simulink model "Pendulum02"  (R2018a)
settings: Solver=ode15s  StartTime=0.0  StopTime=5  MaxStep=0.001  RelTol=1e-3  EnableMultiTasking=on
values from neighbouring files (symbols this model uses):
  a = 1 / muscle_width^2    (= 3.1887755102)    [OldCodeForComparison.m]    (also in Parameters02.m)
  A0 = 0.2741    [OldCodeForComparison.m]    (also in Parameters02.m)
  A1 = -0.0627    [OldCodeForComparison.m]    (also in Parameters02.m)
  a_rel = 0.41    [OldCodeForComparison.m]    (also in Parameters02.m)
  alpha_a = 0.3 * 5/9    (= 0.166666666667)    [OldCodeForComparison.m]    (also in Parameters02.m)
  alpha_theta = 0.0    (= 0)    [OldCodeForComparison.m]    (also in Parameters02.m)
  alpha_v = 3.0 * 5/9    (= 1.66666666667)    [OldCodeForComparison.m]    (also in Parameters02.m)
  b_rel = 5.2    [OldCodeForComparison.m]    (also in Parameters02.m)
  d_l_CE = 0.06    [OldCodeForComparison.m]    (also in Parameters02.m)
  d_theta = 0.06    [OldCodeForComparison.m]    (also in Parameters02.m)
  d_thetaDot = 0.12    [OldCodeForComparison.m]    (also in Parameters02.m)
  d_thetaTwoDot = 0.12    [OldCodeForComparison.m]    (also in Parameters02.m)
  d_v_CE = 0.03    [OldCodeForComparison.m]    (also in Parameters02.m)
  F_max = 1.0e+04 * (0.5991 + 0.2996)    (= 8987)    [OldCodeForComparison.m]    (also in Parameters02.m)
  h_com = 1    [Parameters02.m]
  K_l = 1.0    (= 1)    [OldCodeForComparison.m]    (also in Parameters02.m)
  K_SE = 1.8e+05    (= 180000)    [OldCodeForComparison.m]    (also in Parameters02.m)
  K_v = 0.3    [OldCodeForComparison.m]    (also in Parameters02.m)
  l_CE_init = l_MTC - l_SE    [calculateMuscleEquilibriumState.m]
  l_CE_opt = 0.055    [OldCodeForComparison.m]    (also in Parameters02.m)
  l_SE_0 = 0.2356    [OldCodeForComparison.m]    (also in Parameters02.m)
  lambda_init = l_CE_init - 1 / K_l * STIM_init    [calculateMuscleEquilibriumState.m]
  m_body = 80    [Parameters02.m]
  muscle_c = 1.3700e-04    (= 0.000137)    [OldCodeForComparison.m]    (also in Parameters02.m)
  muscle_eta = 52700    [OldCodeForComparison.m]    (also in Parameters02.m)
  muscle_k = 2.9    [OldCodeForComparison.m]    (also in Parameters02.m)
  muscle_m = 11.3    [OldCodeForComparison.m]    (also in Parameters02.m)
  muscle_q0 = 0.005    [OldCodeForComparison.m]    (also in Parameters02.m)
  q_0 = 5e-03    (= 0.005)    [OldCodeForComparison.m]    (also in Parameters02.m)
  q_crit = 0.03    [OldCodeForComparison.m]    (also in Parameters02.m)
  theta_init = -0.05    [OldCodeForComparison.m]    (also in Parameters02.m)
undefined symbols (not defined in the file or in its folder): X, Y, Z
libraries: sm_lib x10, nesl_utility x9
settings Model: Creator=reimajbi  LastModifiedBy=reimajbi
settings DataIOCC: LimitDataPoints=on
settings OptimizationCC: LifeSpan=inf
settings DebuggingCC: AllowSymbolicDim=off  SFUnexpectedBacktrackingDiag=warning  SFNoUnconditionalDefaultTransitionDiag=warning  SFExecutionAtInitializationDiag=none
settings CodeAppCC: StateflowObjectComments=on
settings GRTTargetCC: TargetLangStandard=C89/C90 (ANSI)  GeneratePreprocessorConditionals=Disable all
settings ConfigComp: CovMetricSettings=dw  CovHtmlReporting=on  CovSaveCumulativeToWorkspaceVar=on  CovSaveSingleToWorkspaceVar=on  CovExternalEMLEnable=off  CovSFcnEnable=off
settings SimscapeCC: SimscapeNominalValues="[{\"value\":\"10\",\"unit\":\"V\"},{\"value\":\"1\",\"unit\":\"A\"},{\"value\":\"10\",\"unit\":\"N*m\"},{\"value\":\"10\",\"unit\":\"bar\"},{\"value\":\"100\",\"unit\":\"kJ/kg\"},{\"value\":\"1\",\"unit\":\"kW\"},{\"value\":\"300\",\"unit\":\"K\"},{\"value\":\"100\",\"unit\":\"cm^3/s\"},{\"value\":\"1\",\"unit\":\"kN\"},{\"value\":\"1\",\"unit\":\"g/cm^3\"},{\"value\":\"1\",\"unit\":\"l\"},{\"value\":\"1\",\"unit\":\"cm^2\"},{\"value\":\"60\",\"unit\":\"Hz\"}]"  SimscapeLogType=all  SimscapeLogDataHistory=10000
settings ConfigurationSet: Description=SimMechanics 2G

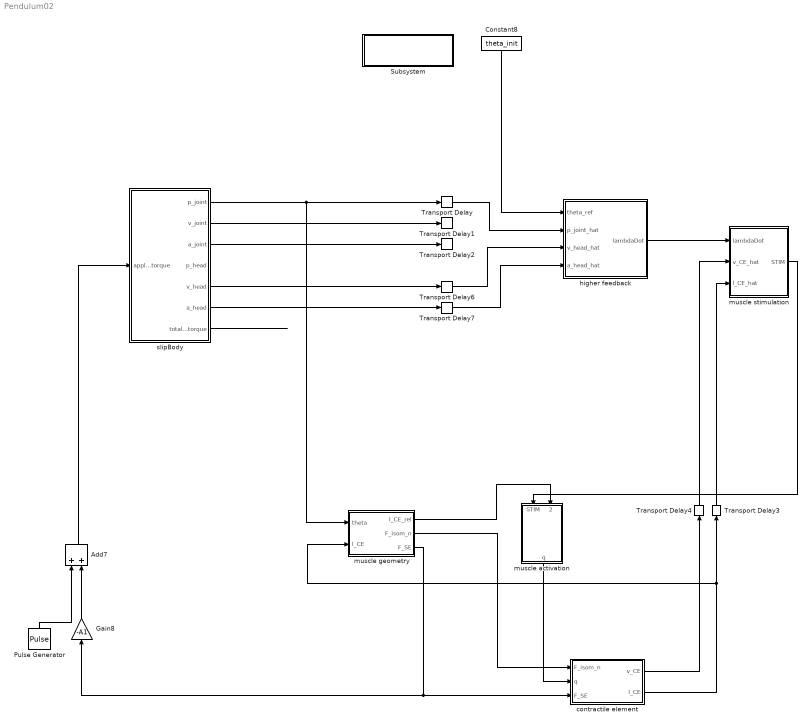
== system Pendulum02 ==
  Add7 : Sum
  Constant8 : Constant  Value=theta_init
  Gain8 : Gain  Gain=-A1
  Pulse Generator : DiscretePulseGenerator  PulseType=Time based  Amplitude=-50  Period=100  PulseWidth=0.2  PhaseDelay=0.1
  Subsystem : Subsystem
      settings: OpenFcn=open_system('sm_lib')
      mask Display: disp(sprintf('Open Simscape Multibody\nLibrary'));
  Transport Delay : TransportDelay  DelayTime=d_theta  InitialOutput=theta_init
  Transport Delay1 : TransportDelay  DelayTime=d_thetaDot
  Transport Delay2 : TransportDelay  DelayTime=d_thetaTwoDot
  Transport Delay3 : TransportDelay  DelayTime=d_l_CE  InitialOutput=l_CE_init
  Transport Delay4 : TransportDelay  DelayTime=d_v_CE
  Transport Delay6 : TransportDelay  DelayTime=d_thetaDot
  Transport Delay7 : TransportDelay  DelayTime=d_thetaTwoDot
  contractile element : Subsystem
  higher feedback : Subsystem
  muscle activation : Subsystem
  muscle geometry : Subsystem
  muscle stimulation : Subsystem
  slipBody : Subsystem  TreatAsAtomicUnit=on
  wires:
  Pulse Generator/1 -> Add7/1
  Gain8/1 -> Add7/2
  contractile element/1(v_CE) -> Transport Delay4/1
  contractile element/2(l_CE) -> muscle geometry/2(l_CE), Transport Delay3/1
  muscle activation/1(q) -> contractile element/2(q)
  Constant8/1 -> higher feedback/1(theta_ref)
  Transport Delay/1 -> higher feedback/2(p_joint_hat)
  Transport Delay6/1 -> higher feedback/3(v_head_hat)
  Transport Delay7/1 -> higher feedback/4(a_head_hat)
  higher feedback/1(lambdaDot) -> muscle stimulation/1(lambdaDot)
  Transport Delay4/1 -> muscle stimulation/2(v_CE_hat)
  Transport Delay3/1 -> muscle stimulation/3(l_CE_hat)
  muscle stimulation/1(STIM) -> muscle activation/1(STIM)
  muscle geometry/3(F_SE) -> Gain8/1, contractile element/3(F_SE)
  muscle geometry/1(l_CE_rel) -> muscle activation/2(l_CE_rel)
  muscle geometry/2(F_isom_n) -> contractile element/1(F_isom_n)
  slipBody/1(p_joint) -> muscle geometry/1(theta), Transport Delay/1
  Add7/1 -> slipBody/1(applied_torque)
  slipBody/2(v_joint) -> Transport Delay1/1
  slipBody/3(a_joint) -> Transport Delay2/1
  slipBody/5(v_head) -> Transport Delay6/1
  slipBody/6(a_head) -> Transport Delay7/1
  slipBody/7(total_torque) -> ?

== system Pendulum02/Subsystem ==

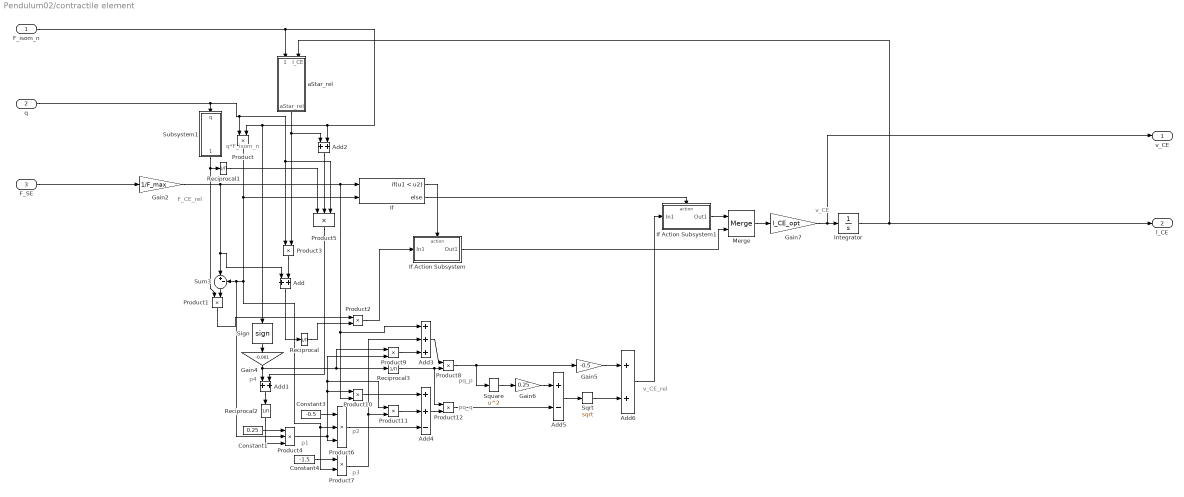
== system Pendulum02/contractile element ==
  note: v_CE_rel
  note: pq_q
  note: F_CE_rel
  note: p3
  note: p2
  note: q*F_isom_n
  note: p1
  note: p4
  note: pq_p
  note: v_CE
  F_isom_n : Inport
  q : Inport  Port=2
  F_SE : Inport  Port=3
  Add{,1..2,6} (4 alike) : Sum
  Add3 : Sum  Inputs=+++
  Add4 : Sum  Inputs=++-
  Add5 : Sum  Inputs=+-
  Constant1 : Constant  Value=0.25
  Constant3 : Constant  Value=-0.5
  Constant4 : Constant  Value=-1.5
  Gain2 : Gain  Gain=1/F_max
  Gain4 : Gain  Gain=-0.001
  Gain5 : Gain  Gain=-0.5
  Gain6 : Gain  Gain=0.25
  Gain7 : Gain  Gain=l_CE_opt
  If : If  NumInputs=2  IfExpression=u1 < u2
  If Action Subsystem : Subsystem  TreatAsAtomicUnit=on
  If Action Subsystem1 : Subsystem  TreatAsAtomicUnit=on
  Integrator : Integrator  InitialCondition=l_CE_init
  Merge : Merge
  Product{,1..3,7..12} (10 alike) : Product
  Product4 : Product  Inputs=3
  Product5 : Product  Inputs=3
  Product6 : Product  Inputs=3
  Reciprocal{,1..3} (4 alike) : Product  Inputs=/
  Sign : Signum
  Sqrt : Sqrt  SaturateOnIntegerOverflow=on
  Square : Math  Operator=square  SaturateOnIntegerOverflow=on
  Subsystem1 : Subsystem
  Sum3 : Sum  Inputs=|+-
  aStar_rel : Subsystem
  v_CE : Outport
  l_CE : Outport  Port=2
  wires:
  Sqrt/1 -> Add6/2
  Product1/1 -> Product2/1
  Add5/1 -> Sqrt/1
  Product10/1 -> Add4/1
  Constant1/1 -> Product4/1
  Gain6/1 -> Add5/1
  Add3/1 -> Product8/1
  Product5/1 -> Add1/2
  Product9/1 -> Add3/3
  Square/1 -> Gain6/1
  Add4/1 -> Product12/2
  F_SE/1 -> Gain2/1
  Reciprocal1/1 -> Product5/1
  Add2/1 -> Product5/2
  Reciprocal/1 -> Product2/2
  Product3/1 -> Add/2
  If Action Subsystem1/1(Out1) -> Merge/1
  Add1/1 -> Reciprocal2/1
  Sign/1 -> Gain4/1
  Product7/1 -> Add3/2, Product11/2
  Reciprocal3/1 -> Product12/1, Product8/2
  If/1 -> If Action Subsystem/Action
  Product2/1 -> If Action Subsystem/1(In1)
  Product11/1 -> Add4/2
  Gain4/1 -> Product9/1, Reciprocal3/1, Add1/1
  Add6/1 -> If Action Subsystem1/1(In1)
  Add/1 -> Reciprocal/1
  Product12/1 -> Add5/2
  Subsystem1/1(bStar_rel) -> Reciprocal1/1, Product1/1
  q/1 -> Product5/3, Product3/1, Product/1, Subsystem1/1(q)
  Gain7/1 -> v_CE/1, Integrator/1
  Constant4/1 -> Product7/1
  Gain5/1 -> Add6/1
  Product8/1 -> Square/1, Gain5/1
  Gain2/1 -> Sum3/1, Add/1, If/1, Add3/1, Product10/2
  Product4/1 -> Product10/1, Product11/1, Product9/2, Product6/3
  If/2 -> If Action Subsystem1/Action
  Integrator/1 -> l_CE/1, aStar_rel/2(l_CE)
  Sum3/1 -> Product1/2
  aStar_rel/1(aStar_rel) -> Add2/1, Product3/2
  If Action Subsystem/1(Out1) -> Merge/2
  Product6/1 -> Add4/3
  Reciprocal2/1 -> Product4/3
  F_isom_n/1 -> aStar_rel/1(F_isom_n), Sign/1, Product/2, Add2/2
  Constant3/1 -> Product6/1
  Merge/1 -> Gain7/1
  Product/1 -> Product7/2, Product6/2, Product4/2, Sum3/2, If/2

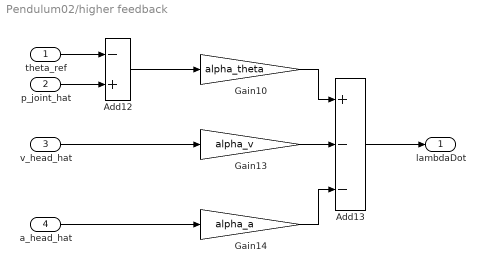
== system Pendulum02/higher feedback ==
  theta_ref : Inport
  p_joint_hat : Inport  Port=2
  v_head_hat : Inport  Port=3
  a_head_hat : Inport  Port=4
  Add12 : Sum  Inputs=-+
  Add13 : Sum  Inputs=+--
  Gain10 : Gain  Gain=alpha_theta
  Gain13 : Gain  Gain=alpha_v
  Gain14 : Gain  Gain=alpha_a
  lambdaDot : Outport
  wires:
  Add13/1 -> lambdaDot/1
  a_head_hat/1 -> Gain14/1
  v_head_hat/1 -> Gain13/1
  Gain10/1 -> Add13/1
  Gain14/1 -> Add13/3
  Gain13/1 -> Add13/2
  p_joint_hat/1 -> Add12/2
  theta_ref/1 -> Add12/1
  Add12/1 -> Gain10/1

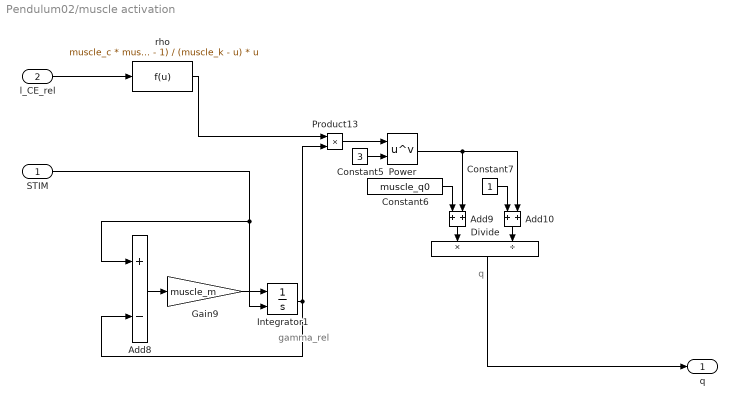
== system Pendulum02/muscle activation ==
  note: gamma_rel
  note: q
  STIM : Inport
  l_CE_rel : Inport  Port=2
  Add10 : Sum
  Add8 : Sum  Inputs=+-
  Add9 : Sum
  Constant5 : Constant  Value=3
  Constant6 : Constant  Value=muscle_q0
  Constant7 : Constant
  Divide : Product  Inputs=*/
  Gain9 : Gain  Gain=muscle_m
  Integrator1 : Integrator  InitialConditionSource=external  InitialCondition=0.038159574513235
  Power : Math  Operator=pow  SaturateOnIntegerOverflow=on
  Product13 : Product
  rho : Fcn  Expr=muscle_c * muscle_eta * (muscle_k - 1) / (muscle_k - u) * u
  q : Outport
  wires:
  l_CE_rel/1 -> rho/1
  Divide/1 -> q/1
  Constant7/1 -> Add10/1
  Product13/1 -> Power/1
  Constant5/1 -> Power/2
  Gain9/1 -> Integrator1/1
  Constant6/1 -> Add9/1
  Integrator1/1 -> Product13/2, Add8/2
  rho/1 -> Product13/1
  Add9/1 -> Divide/1
  Add10/1 -> Divide/2
  STIM/1 -> Integrator1/2, Add8/1
  Power/1 -> Add9/2, Add10/2
  Add8/1 -> Gain9/1

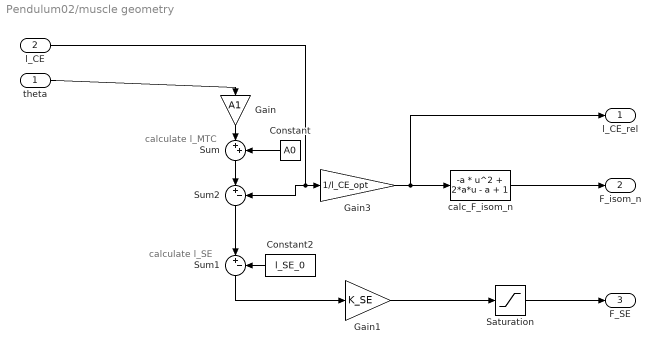
== system Pendulum02/muscle geometry ==
  note: calculate l_MTC
  note: calculate l_SE
  theta : Inport
  l_CE : Inport  Port=2
  Constant : Constant  Value=A0
  Constant2 : Constant  Value=l_SE_0
  Gain : Gain  Gain=A1
  Gain1 : Gain  Gain=K_SE
  Gain3 : Gain  Gain=1/l_CE_opt
  Saturation : Saturate  UpperLimit=inf  LowerLimit=0
  Sum : Sum  Inputs=|++
  Sum1 : Sum  Inputs=|+-
  Sum2 : Sum  Inputs=|+-
  calc_F_isom_n : Fcn  Expr=-a * u^2 + 2*a*u - a + 1
  l_CE_rel : Outport
  F_isom_n : Outport  Port=2
  F_SE : Outport  Port=3
  wires:
  calc_F_isom_n/1 -> F_isom_n/1
  Gain1/1 -> Saturation/1
  Constant/1 -> Sum/2
  Sum/1 -> Sum2/1
  Constant2/1 -> Sum1/2
  l_CE/1 -> Sum2/2, Gain3/1
  Gain3/1 -> l_CE_rel/1, calc_F_isom_n/1
  Sum1/1 -> Gain1/1
  Gain/1 -> Sum/1
  theta/1 -> Gain/1
  Saturation/1 -> F_SE/1
  Sum2/1 -> Sum1/1

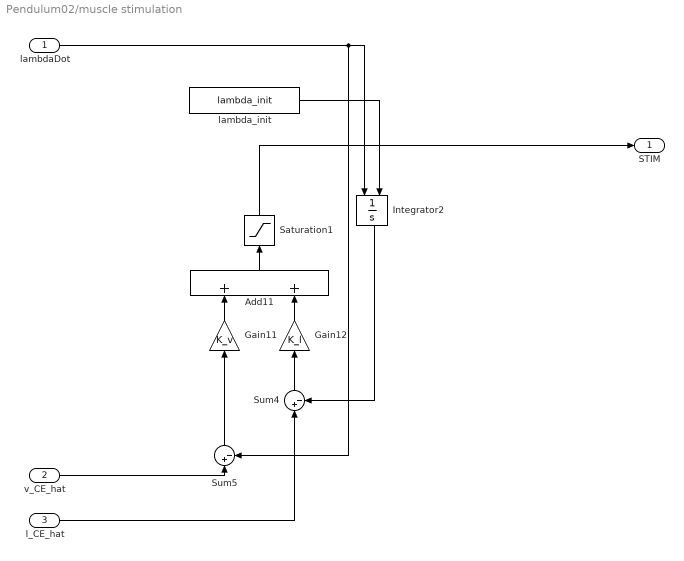
== system Pendulum02/muscle stimulation ==
  lambdaDot : Inport
  v_CE_hat : Inport  Port=2
  l_CE_hat : Inport  Port=3
  Add11 : Sum
  Gain11 : Gain  Gain=K_v
  Gain12 : Gain  Gain=K_l
  Integrator2 : Integrator  InitialConditionSource=external  InitialCondition=0.038159574513235
  Saturation1 : Saturate  UpperLimit=1  LowerLimit=0
  Sum4 : Sum  Inputs=|+-
  Sum5 : Sum  Inputs=|+-
  lambda_init : Constant  Value=lambda_init
  STIM : Outport
  wires:
  Saturation1/1 -> STIM/1
  l_CE_hat/1 -> Sum4/1
  lambda_init/1 -> Integrator2/2
  Sum4/1 -> Gain12/1
  Gain12/1 -> Add11/2
  Sum5/1 -> Gain11/1
  lambdaDot/1 -> Integrator2/1, Sum5/2
  Gain11/1 -> Add11/1
  v_CE_hat/1 -> Sum5/1
  Add11/1 -> Saturation1/1
  Integrator2/1 -> Sum4/2

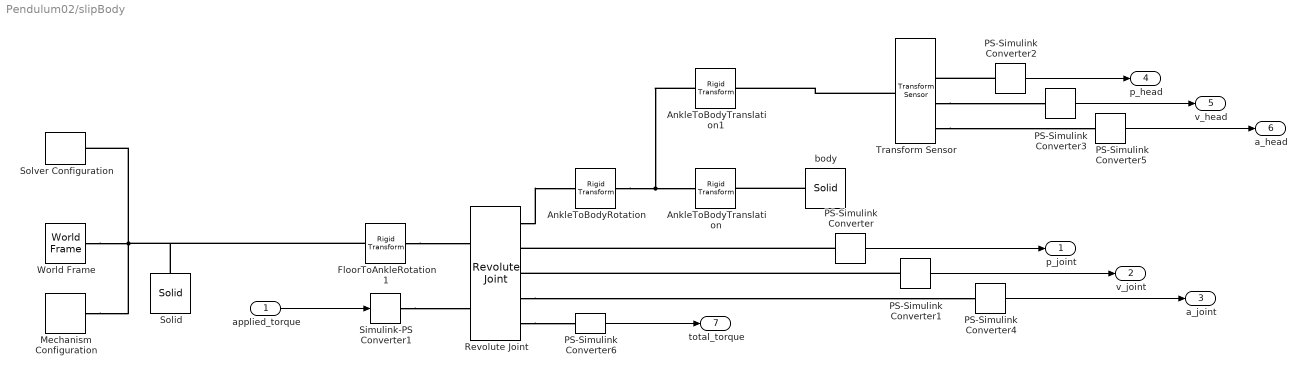
== system Pendulum02/slipBody ==
  applied_torque : Inport
  AnkleToBodyRotation : sm_lib/Frames and Transforms/Rigid Transform  TranslationMethod=None  TranslationStandardOffset=0  TranslationLengthUnit=m  TranslationStandardAxis=+Z  TranslationCartesianOffset=[0 0 0]  TranslationROffset=0  TranslationROffsetUnits=m  TranslationZOffset=0  TranslationZOffsetUnits=m  TranslationThetaOffset=0  TranslationThetaOffsetUnits=deg  RotationMethod=AlignedAxes  RotationAngleUnits=deg  RotationStandardAxis=+Z  RotationAngle=0.0  RotationArbitraryAxis=[0 0 1]  FollAlignAxisA=+Z  BaseAlignAxisA=+X  FollAlignAxisB=+Y  BaseAlignAxisB=+Z  RotationSequenceAxes=FollowerAxes  RotationSequence=XYX  RotationSequenceAngles=[0 0 0]  RotationSequenceAnglesUnits=deg  RotationMatrix=[1 0 0; 0 1 0; 0 0 1]
  AnkleToBodyTranslation : sm_lib/Frames and Transforms/Rigid Transform  TranslationMethod=StandardAxis  TranslationStandardOffset=h_com  TranslationLengthUnit=m  TranslationStandardAxis=+Z  TranslationCartesianOffset=[0 0 0]  TranslationROffset=0  TranslationROffsetUnits=m  TranslationZOffset=0  TranslationZOffsetUnits=m  TranslationThetaOffset=0  TranslationThetaOffsetUnits=deg  RotationMethod=None  RotationAngleUnits=deg  RotationStandardAxis=+Z  RotationAngle=0.0  RotationArbitraryAxis=[0 0 1]  FollAlignAxisA=+X  BaseAlignAxisA=+Y  FollAlignAxisB=+Y  BaseAlignAxisB=+Z  RotationSequenceAxes=FollowerAxes  RotationSequence=XYX  RotationSequenceAngles=[0 0 0]  RotationSequenceAnglesUnits=deg  RotationMatrix=[1 0 0; 0 1 0; 0 0 1]
  AnkleToBodyTranslation1 : sm_lib/Frames and Transforms/Rigid Transform  TranslationMethod=StandardAxis  TranslationStandardOffset=h_head  TranslationLengthUnit=m  TranslationStandardAxis=+Z  TranslationCartesianOffset=[0 0 0]  TranslationROffset=0  TranslationROffsetUnits=m  TranslationZOffset=0  TranslationZOffsetUnits=m  TranslationThetaOffset=0  TranslationThetaOffsetUnits=deg  RotationMethod=None  RotationAngleUnits=deg  RotationStandardAxis=+Z  RotationAngle=0.0  RotationArbitraryAxis=[0 0 1]  FollAlignAxisA=+X  BaseAlignAxisA=+Y  FollAlignAxisB=+Y  BaseAlignAxisB=+Z  RotationSequenceAxes=FollowerAxes  RotationSequence=XYX  RotationSequenceAngles=[0 0 0]  RotationSequenceAnglesUnits=deg  RotationMatrix=[1 0 0; 0 1 0; 0 0 1]
  FloorToAnkleRotation1 : sm_lib/Frames and Transforms/Rigid Transform  TranslationMethod=None  TranslationStandardOffset=0  TranslationLengthUnit=m  TranslationStandardAxis=+Z  TranslationCartesianOffset=[0 0 0]  TranslationROffset=0  TranslationROffsetUnits=m  TranslationZOffset=0  TranslationZOffsetUnits=m  TranslationThetaOffset=0  TranslationThetaOffsetUnits=deg  RotationMethod=AlignedAxes  RotationAngleUnits=deg  RotationStandardAxis=+Z  RotationAngle=0.0  RotationArbitraryAxis=[0 0 1]  FollAlignAxisA=+X  BaseAlignAxisA=+Z  FollAlignAxisB=+Z  BaseAlignAxisB=+Y  RotationSequenceAxes=FollowerAxes  RotationSequence=XYX  RotationSequenceAngles=[0 0 0]  RotationSequenceAnglesUnits=deg  RotationMatrix=[1 0 0; 0 1 0; 0 0 1]
  Mechanism Configuration : sm_lib/Utilities/Mechanism Configuration  UniformGravity=Constant  GravityVector=[0 0 -9.80665]  GravityUnits=m/s^2  LinearizationDelta=0.001
  PS-Simulink Converter{,1..6} (7 alike) : nesl_utility/PS-Simulink Converter  PhysicalDomain=network_engine_domain  SubClassName=ps_output  LeftPortType=input  RightPortType=output  PseudoPeriodic=off  Frequencies=[]  Unit=1  AffineConversion=off
  Revolute Joint : sm_lib/Joints/Revolute Joint  SenseConstraintForce=off  SenseConstraintForceX=off  SenseConstraintForceY=off  SenseConstraintForceZ=off  SenseConstraintTorque=off  SenseConstraintTorqueX=off  SenseConstraintTorqueY=off  SenseConstraintTorqueZ=off  SenseTotalForce=off  SenseTotalForceX=off  SenseTotalForceY=off  SenseTotalForceZ=off  SenseTotalTorque=on  SenseTotalTorqueX=off  SenseTotalTorqueY=off  SenseTotalTorqueZ=off  CompositeWrenchDir=FollowerOnBase  CompositeWrenchFrame=BaseFrame  EquilibriumPosition=0  EquilibriumPositionUnits=deg  SpringStiffness=0  SpringStiffnessUnits=N*m/deg  DampingCoefficient=0  DampingCoefficientUnits=N*m/(deg/s)  TorqueActuationMode=InputTorque  MotionActuationMode=ComputedMotion  SensePosition=on  SenseVelocity=on  SenseAcceleration=on  SenseTorqueForce=off  PositionTargetSpecify=on  PositionTargetPriority=High  PositionTargetValue=theta_init  PositionTargetValueUnits=rad  VelocityTargetSpecify=off  VelocityTargetPriority=High  VelocityTargetValue=0  VelocityTargetValueUnits=deg/s
  Simulink-PS Converter1 : nesl_utility/Simulink-PS Converter  PhysicalDomain=network_engine_domain  SubClassName=ps_input  LeftPortType=input  RightPortType=output  PseudoPeriodic=off  Frequencies=[]  NoiseDistribution=none  NoiseParameters=[]  Unit=1  AffineConversion=off  FilteringAndDerivatives=zero  SimscapeFilterOrder=1  InputFilterTimeConstant=0.001  UdotUserProvided=1
  Solid : sm_lib/Body Elements/Solid  InertiaType=CalculateFromGeometry  Mass=1  MassUnits=kg  CenterOfMass=[0 0 0]  CenterOfMassUnits=m  MomentsOfInertia=[1 1 1]  MomentsOfInertiaUnits=kg*m^2  ProductsOfInertia=[0 0 0]  ProductsOfInertiaUnits=kg*m^2  DensityBased=on  Density=1000  DensityUnits=kg/m^3  DoExposeReferenceFrame=on  SerializedFrames=<Frames/>  GraphicType=FromGeometry  MarkerShape=Sphere  MarkerSize=10  GraphicVisPropType=SimpleVisualProperties  GraphicDiffuseColor=[0.5 0.5 0.5]  GraphicSpecularColor=[0.5 0.5 0.5 1.0]  GraphicAmbientColor=[0.15 0.15 0.15 1.0]  GraphicEmissiveColor=[0.0 0.0 0.0 1.0]  GraphicShininess=75  GraphicOpacity=1.0  GeometryShape=Brick  RectangleSize=[1 1]  RectangleSizeUnits=m  BrickDimensions=[1 1 0.01]  BrickDimensionUnits=m  CylinderRadius=1  CylinderRadiusUnits=m  CylinderLength=1  CylinderLengthUnits=m  SphereRadius=1  SphereRadiusUnits=m  EllipsoidRadii=[1 1 1]  EllipsoidRadiiUnits=m  ExtrusionCrossSection=[1 1; -1 1; -1 -1; 1 -1]  ExtrusionCrossSectionUnits=m  ExtrusionLength=1  ExtrusionLengthUnits=m  PolygonNumSides=3  PolygonOuterRadius=1  PolygonOuterRadiusUnits=m  ExtGeomFileType=STEP  ExtGeomFileUnits=m  RevolutionCrossSection=[1 1; 1 -1; 2 -1; 2 1]  RevolutionCrossSectionUnits=m  RevolutionExtent=Full  RevolutionAngle=180  RevolutionAngleUnits=deg
  Solver Configuration : nesl_utility/Solver Configuration  PhysicalDomain=network_engine_domain  SubClassName=solver  LeftPortType=input  RightPortType=generic  Tones=[]  Harmonics=[]  SimulateNoise=off  Profile=off  UseLocalSampling=off  EnableSwitchedLinearOptims=on  FrequencyDomain=off  UseCCode=off  RelTol=0.001  AbsTol=1e-06  MinStep=1e-09  ToWorkspace=off  RevertToSquareIcSolve=off  NumHomotopyIterations=100  PhasorMode=off  PhasorModeNumHarmonics=1  DoDC=off  ResidualTolerance=1e-09  UseLocalSolver=off  LocalSolverChoice=NE_BACKWARD_EULER_ADVANCER  LocalSolverSampleTime=0.001  DoFixedCost=off  MaxNonlinIter=3  MaxModeIter=2  LinearAlgebra=Sparse  EquationFormulation=NE_TIME_EF  DelaysMemoryBudget=1024  AutomaticFiltering=on  FilteringTimeConstant=0.001
  Transform Sensor : sm_lib/Frames and Transforms/Transform Sensor  MeasurementFrame=World  SenseAngle=off  SenseAxis=off  SenseAngle1=off  SenseAngle2=off  SenseAngle3=off  SenseQ=off  SenseR=off  SenseOmegaX=off  SenseOmegaY=off  SenseOmegaZ=off  SenseOmega1=off  SenseOmega2=off  SenseOmega3=off  SenseQDot=off  SenseRDot=off  SenseAlphaX=off  SenseAlphaY=off  SenseAlphaZ=off  SenseAlpha1=off  SenseAlpha2=off  SenseAlpha3=off  SenseQDDot=off  SenseRDDot=off  SenseX=on  SenseY=off  SenseZ=off  SenseRad=off  SenseAzim=off  SenseDist=off  SenseInc=off  SenseXDot=on  SenseYDot=off  SenseZDot=off  SenseRadDot=off  SenseAzimDot=off  SenseDistDot=off  SenseIncDot=off  SenseXDDot=on  SenseYDDot=off  SenseZDDot=off  SenseRadDDot=off  SenseAzimDDot=off  SenseDistDDot=off  SenseIncDDot=off
  World Frame : sm_lib/Frames and Transforms/World Frame
  body : sm_lib/Body Elements/Solid  InertiaType=Custom  Mass=m_body  MassUnits=kg  CenterOfMass=[0 0 0]  CenterOfMassUnits=m  MomentsOfInertia=[27 27 1]  MomentsOfInertiaUnits=kg*m^2  ProductsOfInertia=[0 0 0]  ProductsOfInertiaUnits=kg*m^2  DensityBased=off  Density=1000  DensityUnits=kg/m^3  DoExposeReferenceFrame=on  SerializedFrames=<Frames/>  GraphicType=FromGeometry  MarkerShape=Sphere  MarkerSize=10  GraphicVisPropType=SimpleVisualProperties  GraphicDiffuseColor=[0.5 0.5 0.5]  GraphicSpecularColor=[0.5 0.5 0.5 1.0]  GraphicAmbientColor=[0.15 0.15 0.15 1.0]  GraphicEmissiveColor=[0.0 0.0 0.0 1.0]  GraphicShininess=75  GraphicOpacity=1.0  GeometryShape=Cylinder  RectangleSize=[1 1]  RectangleSizeUnits=m  BrickDimensions=[1 1 1]  BrickDimensionUnits=cm  CylinderRadius=r_body  CylinderRadiusUnits=m  CylinderLength=h_com*2  CylinderLengthUnits=m  SphereRadius=1  SphereRadiusUnits=m  EllipsoidRadii=[1 1 1]  EllipsoidRadiiUnits=m  ExtrusionCrossSection=[1 1; -1 1; -1 -1; 1 -1]  ExtrusionCrossSectionUnits=m  ExtrusionLength=1  ExtrusionLengthUnits=m  PolygonNumSides=3  PolygonOuterRadius=1  PolygonOuterRadiusUnits=m  ExtGeomFileType=STEP  ExtGeomFileUnits=m  RevolutionCrossSection=[1 1; 1 -1; 2 -1; 2 1]  RevolutionCrossSectionUnits=m  RevolutionExtent=Full  RevolutionAngle=180  RevolutionAngleUnits=deg
  p_joint : Outport
  v_joint : Outport  Port=2
  a_joint : Outport  Port=3
  p_head : Outport  Port=4
  v_head : Outport  Port=5
  a_head : Outport  Port=6
  total_torque : Outport  Port=7
  wires:
  PS-Simulink Converter1/1 -> v_joint/1
  PS-Simulink Converter/1 -> p_joint/1
  PS-Simulink Converter6/1 -> total_torque/1
  PS-Simulink Converter4/1 -> a_joint/1
  applied_torque/1 -> Simulink-PS Converter1/1
  PS-Simulink Converter5/1 -> a_head/1
  PS-Simulink Converter3/1 -> v_head/1
  PS-Simulink Converter2/1 -> p_head/1
  connections:
  Revolute Joint/RConn5 -- PS-Simulink Converter6/LConn1
  Transform Sensor/LConn1 -- AnkleToBodyTranslation1/RConn1
  FloorToAnkleRotation1/RConn1 -- Revolute Joint/LConn1
  PS-Simulink Converter/LConn1 -- Revolute Joint/RConn2
  Revolute Joint/RConn1 -- AnkleToBodyRotation/LConn1
  body/RConn1 -- AnkleToBodyTranslation/RConn1
  Transform Sensor/RConn3 -- PS-Simulink Converter3/LConn1
  Revolute Joint/RConn4 -- PS-Simulink Converter4/LConn1
  Simulink-PS Converter1/RConn1 -- Revolute Joint/LConn2
  PS-Simulink Converter2/LConn1 -- Transform Sensor/RConn2
  Mechanism Configuration/RConn1 -- Solid/RConn1 -- FloorToAnkleRotation1/LConn1 -- World Frame/RConn1 -- Solver Configuration/RConn1
  AnkleToBodyRotation/RConn1 -- AnkleToBodyTranslation1/LConn1 -- AnkleToBodyTranslation/LConn1
  Transform Sensor/RConn4 -- PS-Simulink Converter5/LConn1
  PS-Simulink Converter1/LConn1 -- Revolute Joint/RConn3

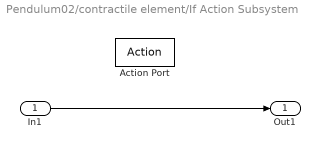
== system Pendulum02/contractile element/If Action Subsystem ==
  In1 : Inport
  Action Port : ActionPort  ActionType=then
  Out1 : Outport
  wires:
  In1/1 -> Out1/1

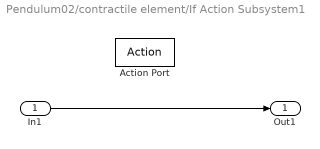
== system Pendulum02/contractile element/If Action Subsystem1 ==
  In1 : Inport
  Action Port : ActionPort  ActionType=else
  Out1 : Outport
  wires:
  In1/1 -> Out1/1

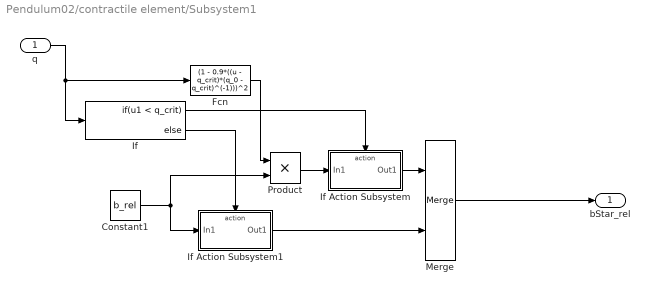
== system Pendulum02/contractile element/Subsystem1 ==
  q : Inport
  Constant1 : Constant  Value=b_rel
  Fcn : Fcn  Expr=(1 - 0.9*((u - q_crit)*(q_0 - q_crit)^(-1)))^2
  If : If  IfExpression=u1 < q_crit
  If Action Subsystem : Subsystem  TreatAsAtomicUnit=on
  If Action Subsystem1 : Subsystem  TreatAsAtomicUnit=on
  Merge : Merge
  Product : Product
  bStar_rel : Outport
  wires:
  Merge/1 -> bStar_rel/1
  If Action Subsystem/1(Out1) -> Merge/1
  If/2 -> If Action Subsystem1/Action
  Constant1/1 -> Product/2, If Action Subsystem1/1(In1)
  q/1 -> Fcn/1, If/1
  Fcn/1 -> Product/1
  Product/1 -> If Action Subsystem/1(In1)
  If/1 -> If Action Subsystem/Action
  If Action Subsystem1/1(Out1) -> Merge/2

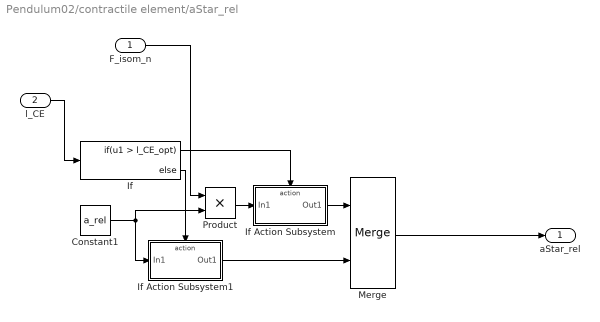
== system Pendulum02/contractile element/aStar_rel ==
  F_isom_n : Inport
  l_CE : Inport  Port=2
  Constant1 : Constant  Value=a_rel
  If : If  IfExpression=u1 > l_CE_opt
  If Action Subsystem : Subsystem  TreatAsAtomicUnit=on
  If Action Subsystem1 : Subsystem  TreatAsAtomicUnit=on
  Merge : Merge
  Product : Product
  aStar_rel : Outport
  wires:
  If Action Subsystem1/1(Out1) -> Merge/2
  Merge/1 -> aStar_rel/1
  Product/1 -> If Action Subsystem/1(In1)
  F_isom_n/1 -> Product/1
  If Action Subsystem/1(Out1) -> Merge/1
  Constant1/1 -> Product/2, If Action Subsystem1/1(In1)
  If/2 -> If Action Subsystem1/Action
  l_CE/1 -> If/1
  If/1 -> If Action Subsystem/Action

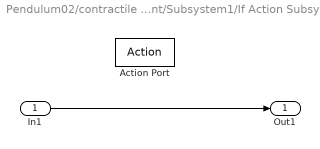
== system Pendulum02/contractile element/Subsystem1/If Action Subsystem ==
  In1 : Inport
  Action Port : ActionPort  ActionType=then
  Out1 : Outport
  wires:
  In1/1 -> Out1/1

== system Pendulum02/contractile element/Subsystem1/If Action Subsystem1 ==
  In1 : Inport
  Action Port : ActionPort  ActionType=else
  Out1 : Outport
  wires:
  In1/1 -> Out1/1

== system Pendulum02/contractile element/aStar_rel/If Action Subsystem ==
  In1 : Inport
  Action Port : ActionPort  ActionType=then
  Out1 : Outport
  wires:
  In1/1 -> Out1/1

== system Pendulum02/contractile element/aStar_rel/If Action Subsystem1 ==
  In1 : Inport
  Action Port : ActionPort  ActionType=else
  Out1 : Outport
  wires:
  In1/1 -> Out1/1
